simulink model "CCC"  (R2024b)
settings: Solver=ode15s  StartTime=0.0  StopTime=10.0  MaxStep=1E-3  RelTol=1e-3
settings Model: Creator=Panzzi  LastModifiedBy=Panzzi
settings DataIOCC: ReturnWorkspaceOutputs=off  TimeSaveName=t
settings DebuggingCC: AlgebraicLoopMsg=none  ArtificialAlgebraicLoopMsg=none  BlockPriorityViolationMsg=error  MinStepSizeMsg=error  MaxConsecutiveZCsMsg=none  OperatingPointInterfaceChecksumMismatchMsg=none

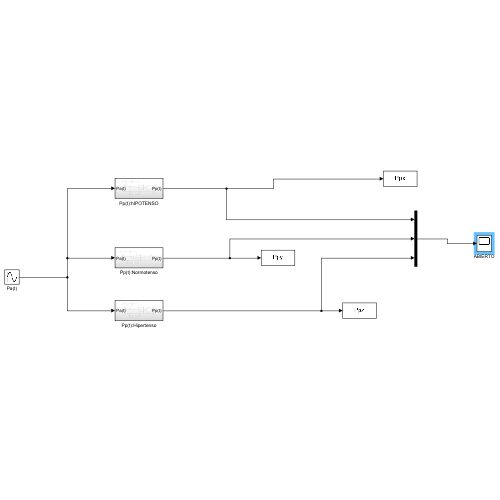
[thumbnail: Simulink's stored preview of the top-level diagram]
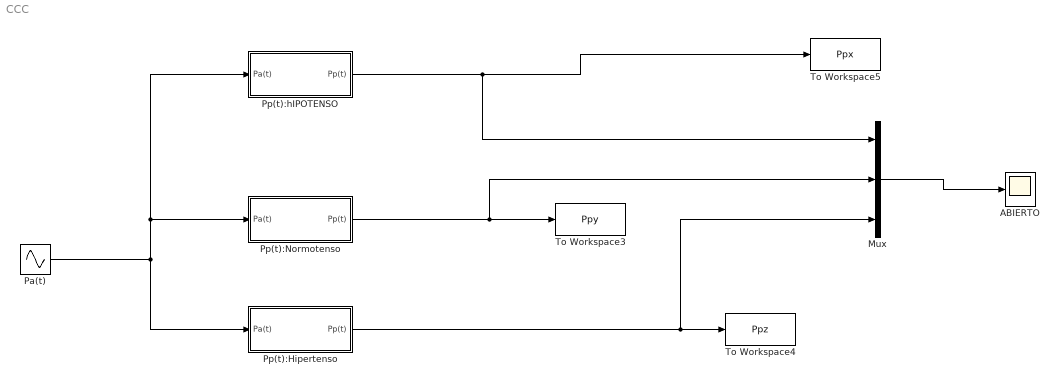
== system CCC ==
  ABIERTO : Scope
  Mux : Mux  Inputs=3
  Pa(t) : Sin  Amplitude=2.5  Frequency=2*pi  SampleTime=0
  Pp(t):Hipertenso : Subsystem
  Pp(t):Normotenso : Subsystem
  Pp(t):hIPOTENSO : Subsystem
  To Workspace3 : ToWorkspace  VariableName=Ppy  SampleTime=-1
  To Workspace4 : ToWorkspace  VariableName=Ppz  SampleTime=-1
  To Workspace5 : ToWorkspace  VariableName=Ppx  SampleTime=-1
  wires:
  Pp(t):Hipertenso/1(Pp(t)) -> Mux/3, To Workspace4/1
  Pa(t)/1 -> Pp(t):Normotenso/1(Pa(t)), Pp(t):hIPOTENSO/1(Pa(t)), Pp(t):Hipertenso/1(Pa(t))
  Pp(t):Normotenso/1(Pp(t)) -> Mux/2, To Workspace3/1
  Pp(t):hIPOTENSO/1(Pp(t)) -> Mux/1, To Workspace5/1
  Mux/1 -> ABIERTO/1

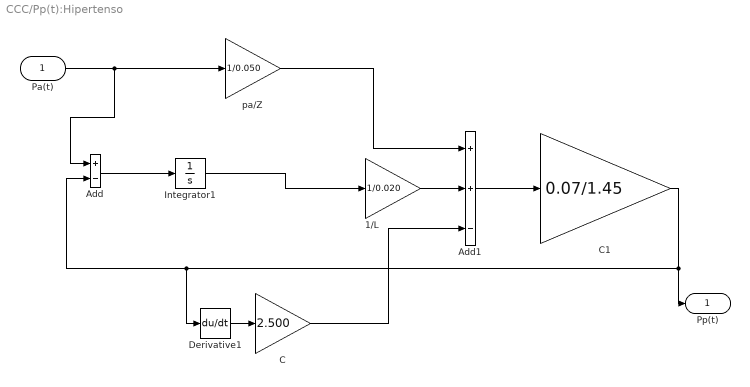
== system CCC/Pp(t):Hipertenso ==
  Pa(t) : Inport
  1/L : Gain  Gain=1/0.020
  Add : Sum  Inputs=+-
  Add1 : Sum  Inputs=++-
  C : Gain  Gain=2.500
  C1 : Gain  Gain=0.07/1.45
  Derivative1 : Derivative
  Integrator1 : Integrator
  pa/Z : Gain  Gain=1/0.050
  Pp(t) : Outport
  wires:
  Pa(t)/1 -> Add/1, pa/Z/1
  C1/1 -> Derivative1/1, Add/2, Pp(t)/1
  Add1/1 -> C1/1
  pa/Z/1 -> Add1/1
  Derivative1/1 -> C/1
  C/1 -> Add1/3
  1/L/1 -> Add1/2
  Integrator1/1 -> 1/L/1
  Add/1 -> Integrator1/1

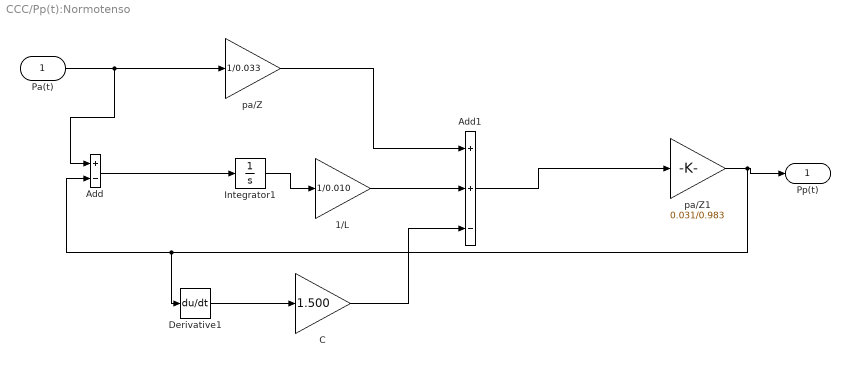
== system CCC/Pp(t):Normotenso ==
  Pa(t) : Inport
  1/L : Gain  Gain=1/0.010
  Add : Sum  Inputs=+-
  Add1 : Sum  Inputs=++-
  C : Gain  Gain=1.500
  Derivative1 : Derivative
  Integrator1 : Integrator
  pa/Z : Gain  Gain=1/0.033
  pa/Z1 : Gain  Gain=0.031/0.983
  Pp(t) : Outport
  wires:
  Pa(t)/1 -> Add/1, pa/Z/1
  Add1/1 -> pa/Z1/1
  pa/Z1/1 -> Derivative1/1, Add/2, Pp(t)/1
  pa/Z/1 -> Add1/1
  1/L/1 -> Add1/2
  Integrator1/1 -> 1/L/1
  Add/1 -> Integrator1/1
  Derivative1/1 -> C/1
  C/1 -> Add1/3

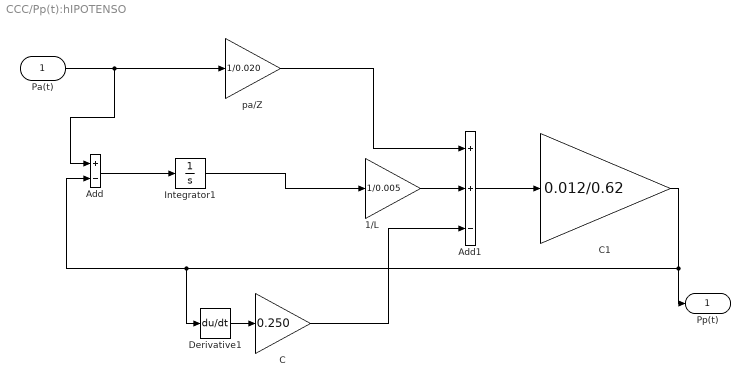
== system CCC/Pp(t):hIPOTENSO ==
  Pa(t) : Inport
  1/L : Gain  Gain=1/0.005
  Add : Sum  Inputs=+-
  Add1 : Sum  Inputs=++-
  C : Gain  Gain=0.250
  C1 : Gain  Gain=0.012/0.62
  Derivative1 : Derivative
  Integrator1 : Integrator
  pa/Z : Gain  Gain=1/0.020
  Pp(t) : Outport
  wires:
  Pa(t)/1 -> Add/1, pa/Z/1
  C1/1 -> Derivative1/1, Add/2, Pp(t)/1
  Add1/1 -> C1/1
  pa/Z/1 -> Add1/1
  Derivative1/1 -> C/1
  C/1 -> Add1/3
  1/L/1 -> Add1/2
  Integrator1/1 -> 1/L/1
  Add/1 -> Integrator1/1
